simulink model "Model_InterpretationEngine64"  (R2022b)
settings: Solver=FixedStepDiscrete  StartTime=0.0  StopTime=5  RelTol=1e-3  EnableMultiTasking=on
InitFcn:
  | % Initialize model
  | ModelSettings=BTConfig.GetModelSettings();
  | 
  | ModelSettings.Validate();
  | 
  | ModelInit;
  | 
  | 
  | % load library data
  | GainLibrary_data;
  | % Load saved values from partition process
  | CapturedConstMask.LoadMapFromFile(bdroot)
  | % Load saved values from partition process
  | TSP_Mask.LoadMapFromFile(bdroot)
StartFcn:
  | % make sure all the simulated RTC requests are found
  | %RTC_SIM_OBJ.ValidateREQs();
undefined symbols (not defined in the file or in its folder): NumHFRefBPF, NumHFRefLPF
libraries: StateVar x112, TSP x56, FeaturePath x24
(part 4 of 5)

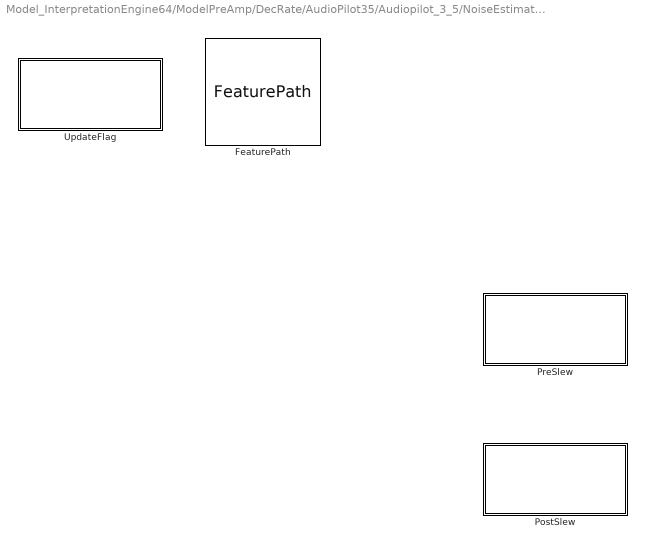
== system Model_InterpretationEngine64/ModelPreAmp/DecRate/AudioPilot35/Audiopilot_3_5/NoiseEstimationVariant/RegularNoiseEstimation/RatioCalculation ==
  FeaturePath : FeaturePath/FeaturePath  FeatureName=Ratio  IsGroup=off  GroupNumber=-1  IsModule=off  TriggerInit=[735 -166 850 -59]
      settings: SourceProductName=Bose Talaria
  PostSlew : Subsystem  mask(Talaria Target State Variable){TriggerInit=[1015 241 1155 309], TspName=PostSlew, StateName=PostSlew, UseSameName=on, IfdefMacro=[]}
      mask prompts: TriggerInit "Hidden: MoveFcn redraw"; TspName "Name:"; StateName "Name of StateVar:"; UseSameName "Use same name for state variable and TSP"; IfdefMacro "Additional #ifdef macro to enable trigger capture:"
      mask help: The TargetStateVar block encapsultes a Target State Probe (TSP), a State Variable, and a Trivial Interpretation between them.
      mask init:
      | [ok,tspPath,activeStatePath] = TargetStateVarMask.Init(gcbh);
      settings: MoveFcn=TargetStateVarMask.CB_TriggerInit(gcbh);
      mask Help: See help for StateVar and TSP blocks
      mask Callback TriggerInit: TargetStateVarMask.CB_TriggerInit(gcbh);
      mask TypeOptions TspName: TSP/TspName
      mask TypeOptions StateName: StateVar/StateName
      mask Callback UseSameName: TargetStateVarMask.CB_UseSameName(gcbh);
      mask TypeOptions IfdefMacro: TSP/IfdefMacro
      mask DialogControl AdvancedPanel Prompt: Advanced
      mask DialogControl ConvertToFullInterpretation Prompt: Irreversible conversion to full interpretation
      mask DialogControl ConvertToFullInterpretation Callback: TargetStateVarMask.CB_ConvertToFullInterpretation(gcbh);
      mask DialogControl ErrorContainer Prompt: Error Messages
      mask DialogControl ErrorText Prompt: The interpreted StateVar value is not yet available
      mask DialogControl TspPathText Prompt: TSP: Current parameter name: [AudiopilotRatioPostSlew]
      mask Display:
      | % retrieve icon definition
      | [path,w,h] = TargetStateVarMask.Icon();
      | 
      | % retrieve the block's pixel size
      | pos = get(gcbh,'position');
      | bw = pos(3) - pos(1);
      | bh = pos(4) - pos(2);
      | 
      | % draw centered icon
      | xAdj = bw/2 - w/2 + 5;
      | yAdj = bh/2 - h/2 + 4;
      | for i=1:length(path)
      | 	patch(path(i).x+xAdj, path(i).y+yAdj, path(i).rgb);
      | end
      | 
      | % show the top name or an X
      | if (exist('ok','var') && ok)
      | 	text(bw*0.5, bh*0.2, tspPath, 'horizontalAlignment', 'center');
      | 	patch(0,0,[1 1 1]);
      | 	patch(bw,bh,[1 1 1]);
      | else
      | 	tx=bw*0.03;
      | 	ty=bh*0.03;
      | 	patch([0 tx bw bw-tx], [ty 0 bh-ty bh], [1 0 0]);
      | 	patch([0 bw-tx bw tx], [bh-ty 0 ty bh], [1 0 0]);
      | end
  PreSlew : Subsystem  mask(Talaria Target State Variable){TriggerInit=[1015 91 1155 159], TspName=PreSlew, StateName=PreSlew, UseSameName=on, IfdefMacro=[]}
      mask prompts: TriggerInit "Hidden: MoveFcn redraw"; TspName "Name:"; StateName "Name of StateVar:"; UseSameName "Use same name for state variable and TSP"; IfdefMacro "Additional #ifdef macro to enable trigger capture:"
      mask help: The TargetStateVar block encapsultes a Target State Probe (TSP), a State Variable, and a Trivial Interpretation between them.
      mask init:
      | [ok,tspPath,activeStatePath] = TargetStateVarMask.Init(gcbh);
      settings: MoveFcn=TargetStateVarMask.CB_TriggerInit(gcbh);
      mask Help: See help for StateVar and TSP blocks
      mask Callback TriggerInit: TargetStateVarMask.CB_TriggerInit(gcbh);
      mask TypeOptions TspName: TSP/TspName
      mask TypeOptions StateName: StateVar/StateName
      mask Callback UseSameName: TargetStateVarMask.CB_UseSameName(gcbh);
      mask TypeOptions IfdefMacro: TSP/IfdefMacro
      mask DialogControl AdvancedPanel Prompt: Advanced
      mask DialogControl ConvertToFullInterpretation Prompt: Irreversible conversion to full interpretation
      mask DialogControl ConvertToFullInterpretation Callback: TargetStateVarMask.CB_ConvertToFullInterpretation(gcbh);
      mask DialogControl ErrorContainer Prompt: Error Messages
      mask DialogControl ErrorText Prompt: The interpreted StateVar value is not yet available
      mask DialogControl TspPathText Prompt: TSP: Current parameter name: [AudiopilotRatioPreSlew]
      mask Display:
      | % retrieve icon definition
      | [path,w,h] = TargetStateVarMask.Icon();
      | 
      | % retrieve the block's pixel size
      | pos = get(gcbh,'position');
      | bw = pos(3) - pos(1);
      | bh = pos(4) - pos(2);
      | 
      | % draw centered icon
      | xAdj = bw/2 - w/2 + 5;
      | yAdj = bh/2 - h/2 + 4;
      | for i=1:length(path)
      | 	patch(path(i).x+xAdj, path(i).y+yAdj, path(i).rgb);
      | end
      | 
      | % show the top name or an X
      | if (exist('ok','var') && ok)
      | 	text(bw*0.5, bh*0.2, tspPath, 'horizontalAlignment', 'center');
      | 	patch(0,0,[1 1 1]);
      | 	patch(bw,bh,[1 1 1]);
      | else
      | 	tx=bw*0.03;
      | 	ty=bh*0.03;
      | 	patch([0 tx bw bw-tx], [ty 0 bh-ty bh], [1 0 0]);
      | 	patch([0 bw-tx bw tx], [bh-ty 0 ty bh], [1 0 0]);
      | end
  UpdateFlag : Subsystem  mask(Talaria Target State Variable){TriggerInit=[550 -144 690 -76], TspName=UpdateFlag, StateName=UpdateFlag, UseSameName=on, IfdefMacro=[]}
      mask prompts: TriggerInit "Hidden: MoveFcn redraw"; TspName "Name:"; StateName "Name of StateVar:"; UseSameName "Use same name for state variable and TSP"; IfdefMacro "Additional #ifdef macro to enable trigger capture:"
      mask help: The TargetStateVar block encapsultes a Target State Probe (TSP), a State Variable, and a Trivial Interpretation between them.
      mask init:
      | [ok,tspPath,activeStatePath] = TargetStateVarMask.Init(gcbh);
      settings: MoveFcn=TargetStateVarMask.CB_TriggerInit(gcbh);
      mask Help: See help for StateVar and TSP blocks
      mask Callback TriggerInit: TargetStateVarMask.CB_TriggerInit(gcbh);
      mask TypeOptions TspName: TSP/TspName
      mask TypeOptions StateName: StateVar/StateName
      mask Callback UseSameName: TargetStateVarMask.CB_UseSameName(gcbh);
      mask TypeOptions IfdefMacro: TSP/IfdefMacro
      mask DialogControl AdvancedPanel Prompt: Advanced
      mask DialogControl ConvertToFullInterpretation Prompt: Irreversible conversion to full interpretation
      mask DialogControl ConvertToFullInterpretation Callback: TargetStateVarMask.CB_ConvertToFullInterpretation(gcbh);
      mask DialogControl ErrorContainer Prompt: Error Messages
      mask DialogControl ErrorText Prompt: The interpreted StateVar value is not yet available
      mask DialogControl TspPathText Prompt: TSP: Current parameter name: [AudiopilotRatioUpdateFlag]
      mask Display:
      | % retrieve icon definition
      | [path,w,h] = TargetStateVarMask.Icon();
      | 
      | % retrieve the block's pixel size
      | pos = get(gcbh,'position');
      | bw = pos(3) - pos(1);
      | bh = pos(4) - pos(2);
      | 
      | % draw centered icon
      | xAdj = bw/2 - w/2 + 5;
      | yAdj = bh/2 - h/2 + 4;
      | for i=1:length(path)
      | 	patch(path(i).x+xAdj, path(i).y+yAdj, path(i).rgb);
      | end
      | 
      | % show the top name or an X
      | if (exist('ok','var') && ok)
      | 	text(bw*0.5, bh*0.2, tspPath, 'horizontalAlignment', 'center');
      | 	patch(0,0,[1 1 1]);
      | 	patch(bw,bh,[1 1 1]);
      | else
      | 	tx=bw*0.03;
      | 	ty=bh*0.03;
      | 	patch([0 tx bw bw-tx], [ty 0 bh-ty bh], [1 0 0]);
      | 	patch([0 bw-tx bw tx], [bh-ty 0 ty bh], [1 0 0]);
      | end

== system Model_InterpretationEngine64/ModelPreAmp/DecRate/AudioPilot35/EntertainmentLevelDetection/AudiopilotLevelDetect/Monitor/env ==
  StateVar : StateVar/StateVar  TriggerInit=[490 139 605 201]  StateName=EnvDb
      settings: SourceProductName=Bose Talaria
  TSP : TSP/TSP  TriggerInit=[110 134 215 206]  TspName=EnvDb  IfDefMacro=IfdefMacro  Role=Automatic
      settings: SourceProductName=Bose Talaria
  TrivialInterpretation : StateVar/TrivialInterpretation  TriggerInit=[330 148 380 192]
      settings: SourceProductName=Bose Talaria
  wires:
  TrivialInterpretation/1 -> StateVar/1
  TSP/1 -> TrivialInterpretation/1

== system Model_InterpretationEngine64/ModelPreAmp/DecRate/AudioPilot35/EntertainmentLevelDetection/AudiopilotLevelDetect/Monitor/level ==
  StateVar : StateVar/StateVar  TriggerInit=[490 139 605 201]  StateName=LevelDbspl
      settings: SourceProductName=Bose Talaria
  TSP : TSP/TSP  TriggerInit=[110 134 215 206]  TspName=LevelDbspl  IfDefMacro=IfdefMacro  Role=Automatic
      settings: SourceProductName=Bose Talaria
  TrivialInterpretation : StateVar/TrivialInterpretation  TriggerInit=[330 148 380 192]
      settings: SourceProductName=Bose Talaria
  wires:
  TrivialInterpretation/1 -> StateVar/1
  TSP/1 -> TrivialInterpretation/1

== system Model_InterpretationEngine64/ModelPreAmp/DecRate/AudioPilot35/EntertainmentLevelDetection/DyneqLevelDetect/Monitor/env ==
  StateVar : StateVar/StateVar  TriggerInit=[490 139 605 201]  StateName=EnvDb
      settings: SourceProductName=Bose Talaria
  TSP : TSP/TSP  TriggerInit=[110 134 215 206]  TspName=EnvDb  IfDefMacro=IfdefMacro  Role=Automatic
      settings: SourceProductName=Bose Talaria
  TrivialInterpretation : StateVar/TrivialInterpretation  TriggerInit=[330 148 380 192]
      settings: SourceProductName=Bose Talaria
  wires:
  TrivialInterpretation/1 -> StateVar/1
  TSP/1 -> TrivialInterpretation/1

== system Model_InterpretationEngine64/ModelPreAmp/DecRate/AudioPilot35/EntertainmentLevelDetection/DyneqLevelDetect/Monitor/level ==
  StateVar : StateVar/StateVar  TriggerInit=[490 139 605 201]  StateName=LevelDbspl
      settings: SourceProductName=Bose Talaria
  TSP : TSP/TSP  TriggerInit=[110 134 215 206]  TspName=LevelDbspl  IfDefMacro=IfdefMacro  Role=Automatic
      settings: SourceProductName=Bose Talaria
  TrivialInterpretation : StateVar/TrivialInterpretation  TriggerInit=[330 148 380 192]
      settings: SourceProductName=Bose Talaria
  wires:
  TrivialInterpretation/1 -> StateVar/1
  TSP/1 -> TrivialInterpretation/1

== system Model_InterpretationEngine64/ModelPreAmp/DecRate/Medusa5H1/MedusaHoligram/Medusa5H1 Part 1/CAE Treble Boost/Audio Passthrough ==
  Target StateVar : Subsystem  mask(Talaria Target State Variable){TriggerInit=[235 166 375 234], TspName=DummyState, StateName=DummyState, UseSameName=on, IfdefMacro=[]}
      mask prompts: TriggerInit "Hidden: MoveFcn redraw"; TspName "Name:"; StateName "Name of StateVar:"; UseSameName "Use same name for state variable and TSP"; IfdefMacro "Additional #ifdef macro to enable trigger capture:"
      mask help: The TargetStateVar block encapsultes a Target State Probe (TSP), a State Variable, and a Trivial Interpretation between them.
      mask init:
      | [ok,tspPath,activeStatePath] = TargetStateVarMask.Init(gcbh);
      settings: MoveFcn=TargetStateVarMask.CB_TriggerInit(gcbh);
      mask Help: See help for StateVar and TSP blocks
      mask Callback TriggerInit: TargetStateVarMask.CB_TriggerInit(gcbh);
      mask TypeOptions TspName: TSP/TspName
      mask TypeOptions StateName: StateVar/StateName
      mask Callback UseSameName: TargetStateVarMask.CB_UseSameName(gcbh);
      mask TypeOptions IfdefMacro: TSP/IfdefMacro
      mask DialogControl AdvancedPanel Prompt: Advanced
      mask DialogControl ConvertToFullInterpretation Prompt: Irreversible conversion to full interpretation
      mask DialogControl ConvertToFullInterpretation Callback: TargetStateVarMask.CB_ConvertToFullInterpretation(gcbh);
      mask DialogControl ErrorContainer Prompt: Error Messages
      mask DialogControl ErrorText Prompt: The interpreted StateVar value is not yet available
      mask DialogControl TspPathText Prompt: TSP: Current parameter name: [PreAmpMedusaDummyState]
      mask Display:
      | % retrieve icon definition
      | [path,w,h] = TargetStateVarMask.Icon();
      | 
      | % retrieve the block's pixel size
      | pos = get(gcbh,'position');
      | bw = pos(3) - pos(1);
      | bh = pos(4) - pos(2);
      | 
      | % draw centered icon
      | xAdj = bw/2 - w/2 + 5;
      | yAdj = bh/2 - h/2 + 4;
      | for i=1:length(path)
      | 	patch(path(i).x+xAdj, path(i).y+yAdj, path(i).rgb);
      | end
      | 
      | % show the top name or an X
      | if (exist('ok','var') && ok)
      | 	text(bw*0.5, bh*0.2, tspPath, 'horizontalAlignment', 'center');
      | 	patch(0,0,[1 1 1]);
      | 	patch(bw,bh,[1 1 1]);
      | else
      | 	tx=bw*0.03;
      | 	ty=bh*0.03;
      | 	patch([0 tx bw bw-tx], [ty 0 bh-ty bh], [1 0 0]);
      | 	patch([0 bw-tx bw tx], [bh-ty 0 ty bh], [1 0 0]);
      | end

== system Model_InterpretationEngine64/ModelPreAmp/DecRate/Medusa5H1/MedusaHoligram/Medusa5H1 Part 1/CAE Treble Boost/CAE Treble Boost ==

== system Model_InterpretationEngine64/ModelPreAmp/DecRate/Medusa5H1/MedusaHoligram/Medusa5H1 Part 2/Mono Detector/Mono Detector ==
  Target StateVar : Subsystem  mask(Talaria Target State Variable){TriggerInit=[875 1951 1015 2019], TspName=LevelCenter, StateName=LevelCenter, UseSameName=on, IfdefMacro=[]}
      mask prompts: TriggerInit "Hidden: MoveFcn redraw"; TspName "Name:"; StateName "Name of StateVar:"; UseSameName "Use same name for state variable and TSP"; IfdefMacro "Additional #ifdef macro to enable trigger capture:"
      mask help: The TargetStateVar block encapsultes a Target State Probe (TSP), a State Variable, and a Trivial Interpretation between them.
      mask init:
      | [ok,tspPath,activeStatePath] = TargetStateVarMask.Init(gcbh);
      settings: MoveFcn=TargetStateVarMask.CB_TriggerInit(gcbh);
      mask Help: See help for StateVar and TSP blocks
      mask Callback TriggerInit: TargetStateVarMask.CB_TriggerInit(gcbh);
      mask TypeOptions TspName: TSP/TspName
      mask TypeOptions StateName: StateVar/StateName
      mask Callback UseSameName: TargetStateVarMask.CB_UseSameName(gcbh);
      mask TypeOptions IfdefMacro: TSP/IfdefMacro
      mask DialogControl AdvancedPanel Prompt: Advanced
      mask DialogControl ConvertToFullInterpretation Prompt: Irreversible conversion to full interpretation
      mask DialogControl ConvertToFullInterpretation Callback: TargetStateVarMask.CB_ConvertToFullInterpretation(gcbh);
      mask DialogControl ErrorContainer Prompt: Error Messages
      mask DialogControl ErrorText Prompt: The interpreted StateVar value is not yet available
      mask DialogControl TspPathText Prompt: TSP: Current parameter name: [PreAmpMedusaMonoDetectorLevelCenter]
      mask Display:
      | % retrieve icon definition
      | [path,w,h] = TargetStateVarMask.Icon();
      | 
      | % retrieve the block's pixel size
      | pos = get(gcbh,'position');
      | bw = pos(3) - pos(1);
      | bh = pos(4) - pos(2);
      | 
      | % draw centered icon
      | xAdj = bw/2 - w/2 + 5;
      | yAdj = bh/2 - h/2 + 4;
      | for i=1:length(path)
      | 	patch(path(i).x+xAdj, path(i).y+yAdj, path(i).rgb);
      | end
      | 
      | % show the top name or an X
      | if (exist('ok','var') && ok)
      | 	text(bw*0.5, bh*0.2, tspPath, 'horizontalAlignment', 'center');
      | 	patch(0,0,[1 1 1]);
      | 	patch(bw,bh,[1 1 1]);
      | else
      | 	tx=bw*0.03;
      | 	ty=bh*0.03;
      | 	patch([0 tx bw bw-tx], [ty 0 bh-ty bh], [1 0 0]);
      | 	patch([0 bw-tx bw tx], [bh-ty 0 ty bh], [1 0 0]);
      | end

== system Model_InterpretationEngine64/ModelPreAmp/DecRate/Medusa5H1/MedusaHoligram/Medusa5H1 Part 2/Mono Detector/Target StateVar ==
  StateVar : StateVar/StateVar  TriggerInit=[490 139 605 201]  StateName=IsStereo
      settings: SourceProductName=Bose Talaria
  TSP : TSP/TSP  TriggerInit=[110 134 215 206]  TspName=IsStereo  IfDefMacro=IfdefMacro  Role=Automatic
      settings: SourceProductName=Bose Talaria
  TrivialInterpretation : StateVar/TrivialInterpretation  TriggerInit=[330 148 380 192]
      settings: SourceProductName=Bose Talaria
  wires:
  TrivialInterpretation/1 -> StateVar/1
  TSP/1 -> TrivialInterpretation/1

== system Model_InterpretationEngine64/ModelPreAmp/DecRate/Medusa5H1/MedusaHoligram/Medusa5H1 Part 2/Mono Detector/Target StateVar1 ==
  StateVar : StateVar/StateVar  TriggerInit=[490 139 605 201]  StateName=IsActive
      settings: SourceProductName=Bose Talaria
  TSP : TSP/TSP  TriggerInit=[110 134 215 206]  TspName=IsActive  IfDefMacro=IfdefMacro  Role=Automatic
      settings: SourceProductName=Bose Talaria
  TrivialInterpretation : StateVar/TrivialInterpretation  TriggerInit=[330 148 380 192]
      settings: SourceProductName=Bose Talaria
  wires:
  TrivialInterpretation/1 -> StateVar/1
  TSP/1 -> TrivialInterpretation/1

== system Model_InterpretationEngine64/NEAR/Near1p1/VolumeMute/VolMuteCh1/Ann1NonEntGainCalc/boost/Target StateVar ==
  StateVar : StateVar/StateVar  TriggerInit=[490 139 605 201]  StateName=GetNonEntBoostLeveldB
      settings: SourceProductName=Bose Talaria
  TSP : TSP/TSP  TriggerInit=[110 134 215 206]  TspName=GetNonEntBoostLeveldB  IfDefMacro=IfdefMacro  Role=Automatic
      settings: SourceProductName=Bose Talaria
  TrivialInterpretation : StateVar/TrivialInterpretation  TriggerInit=[330 148 380 192]
      settings: SourceProductName=Bose Talaria
  wires:
  TrivialInterpretation/1 -> StateVar/1
  TSP/1 -> TrivialInterpretation/1

== system Model_InterpretationEngine64/NEAR/Near1p1/VolumeMute/VolMuteCh2/Ann2NonEntGainCalc/boost/Target StateVar ==
  StateVar : StateVar/StateVar  TriggerInit=[490 139 605 201]  StateName=GetNonEntBoostLeveldB
      settings: SourceProductName=Bose Talaria
  TSP : TSP/TSP  TriggerInit=[110 134 215 206]  TspName=GetNonEntBoostLeveldB  IfDefMacro=IfdefMacro  Role=Automatic
      settings: SourceProductName=Bose Talaria
  TrivialInterpretation : StateVar/TrivialInterpretation  TriggerInit=[330 148 380 192]
      settings: SourceProductName=Bose Talaria
  wires:
  TrivialInterpretation/1 -> StateVar/1
  TSP/1 -> TrivialInterpretation/1

== system Model_InterpretationEngine64/NEAR/Near1p1/VolumeMute/VolMuteCh3/Ann3NonEntGainCalc/boost/Target StateVar ==
  StateVar : StateVar/StateVar  TriggerInit=[490 139 605 201]  StateName=GetNonEntBoostLeveldB
      settings: SourceProductName=Bose Talaria
  TSP : TSP/TSP  TriggerInit=[110 134 215 206]  TspName=GetNonEntBoostLeveldB  IfDefMacro=IfdefMacro  Role=Automatic
      settings: SourceProductName=Bose Talaria
  TrivialInterpretation : StateVar/TrivialInterpretation  TriggerInit=[330 148 380 192]
      settings: SourceProductName=Bose Talaria
  wires:
  TrivialInterpretation/1 -> StateVar/1
  TSP/1 -> TrivialInterpretation/1

== system Model_InterpretationEngine64/NEAR/Near1p1/VolumeMute/VolMuteCh4/Ann4NonEntGainCalc/boost/Target StateVar ==
  StateVar : StateVar/StateVar  TriggerInit=[490 139 605 201]  StateName=GetNonEntBoostLeveldB
      settings: SourceProductName=Bose Talaria
  TSP : TSP/TSP  TriggerInit=[110 134 215 206]  TspName=GetNonEntBoostLeveldB  IfDefMacro=IfdefMacro  Role=Automatic
      settings: SourceProductName=Bose Talaria
  TrivialInterpretation : StateVar/TrivialInterpretation  TriggerInit=[330 148 380 192]
      settings: SourceProductName=Bose Talaria
  wires:
  TrivialInterpretation/1 -> StateVar/1
  TSP/1 -> TrivialInterpretation/1

== system Model_InterpretationEngine64/ModelPreAmp/DecRate/AudioPilot35/Audiopilot_3_5/NoiseEstimationVariant/RegularNoiseEstimation/HFNoiseEstimatorCoh/HfNoiseMusicSeparation  ==
  note: Optimization Idea:
      | 1. Use 1-D array to store HALF 3-D GXY matrix, saving 16 KB
  MicPsdLevel : Subsystem
  NoisePsdLevel : Subsystem

== system Model_InterpretationEngine64/ModelPreAmp/DecRate/AudioPilot35/Audiopilot_3_5/NoiseEstimationVariant/RegularNoiseEstimation/HFNoiseEstimatorCoh/PostProcessing ==
  HfImpulseRejection : Subsystem
  PostSlew : Subsystem  mask(Talaria Target State Variable){TriggerInit=[735 161 875 229], TspName=PostSlew, StateName=PostSlew, UseSameName=on, IfdefMacro=[]}
      mask prompts: TriggerInit "Hidden: MoveFcn redraw"; TspName "Name:"; StateName "Name of StateVar:"; UseSameName "Use same name for state variable and TSP"; IfdefMacro "Additional #ifdef macro to enable trigger capture:"
      mask help: The TargetStateVar block encapsultes a Target State Probe (TSP), a State Variable, and a Trivial Interpretation between them.
      mask init:
      | [ok,tspPath,activeStatePath] = TargetStateVarMask.Init(gcbh);
      settings: MoveFcn=TargetStateVarMask.CB_TriggerInit(gcbh);
      mask Help: See help for StateVar and TSP blocks
      mask Callback TriggerInit: TargetStateVarMask.CB_TriggerInit(gcbh);
      mask TypeOptions TspName: TSP/TspName
      mask TypeOptions StateName: StateVar/StateName
      mask Callback UseSameName: TargetStateVarMask.CB_UseSameName(gcbh);
      mask TypeOptions IfdefMacro: TSP/IfdefMacro
      mask DialogControl AdvancedPanel Prompt: Advanced
      mask DialogControl ConvertToFullInterpretation Prompt: Irreversible conversion to full interpretation
      mask DialogControl ConvertToFullInterpretation Callback: TargetStateVarMask.CB_ConvertToFullInterpretation(gcbh);
      mask DialogControl ErrorContainer Prompt: Error Messages
      mask Display:
      | % retrieve icon definition
      | [path,w,h] = TargetStateVarMask.Icon();
      | 
      | % retrieve the block's pixel size
      | pos = get(gcbh,'position');
      | bw = pos(3) - pos(1);
      | bh = pos(4) - pos(2);
      | 
      | % draw centered icon
      | xAdj = bw/2 - w/2 + 5;
      | yAdj = bh/2 - h/2 + 4;
      | for i=1:length(path)
      | 	patch(path(i).x+xAdj, path(i).y+yAdj, path(i).rgb);
      | end
      | 
      | % show the top name or an X
      | if (exist('ok','var') && ok)
      | 	text(bw*0.5, bh*0.2, tspPath, 'horizontalAlignment', 'center');
      | 	patch(0,0,[1 1 1]);
      | 	patch(bw,bh,[1 1 1]);
      | else
      | 	tx=bw*0.03;
      | 	ty=bh*0.03;
      | 	patch([0 tx bw bw-tx], [ty 0 bh-ty bh], [1 0 0]);
      | 	patch([0 bw-tx bw tx], [bh-ty 0 ty bh], [1 0 0]);
      | end
  PreSlew : Subsystem  mask(Talaria Target State Variable){TriggerInit=[735 251 875 319], TspName=PreSlew, StateName=PreSlew, UseSameName=on, IfdefMacro=[]}
      mask prompts: TriggerInit "Hidden: MoveFcn redraw"; TspName "Name:"; StateName "Name of StateVar:"; UseSameName "Use same name for state variable and TSP"; IfdefMacro "Additional #ifdef macro to enable trigger capture:"
      mask help: The TargetStateVar block encapsultes a Target State Probe (TSP), a State Variable, and a Trivial Interpretation between them.
      mask init:
      | [ok,tspPath,activeStatePath] = TargetStateVarMask.Init(gcbh);
      settings: MoveFcn=TargetStateVarMask.CB_TriggerInit(gcbh);
      mask Help: See help for StateVar and TSP blocks
      mask Callback TriggerInit: TargetStateVarMask.CB_TriggerInit(gcbh);
      mask TypeOptions TspName: TSP/TspName
      mask TypeOptions StateName: StateVar/StateName
      mask Callback UseSameName: TargetStateVarMask.CB_UseSameName(gcbh);
      mask TypeOptions IfdefMacro: TSP/IfdefMacro
      mask DialogControl AdvancedPanel Prompt: Advanced
      mask DialogControl ConvertToFullInterpretation Prompt: Irreversible conversion to full interpretation
      mask DialogControl ConvertToFullInterpretation Callback: TargetStateVarMask.CB_ConvertToFullInterpretation(gcbh);
      mask DialogControl ErrorContainer Prompt: Error Messages
      mask Display:
      | % retrieve icon definition
      | [path,w,h] = TargetStateVarMask.Icon();
      | 
      | % retrieve the block's pixel size
      | pos = get(gcbh,'position');
      | bw = pos(3) - pos(1);
      | bh = pos(4) - pos(2);
      | 
      | % draw centered icon
      | xAdj = bw/2 - w/2 + 5;
      | yAdj = bh/2 - h/2 + 4;
      | for i=1:length(path)
      | 	patch(path(i).x+xAdj, path(i).y+yAdj, path(i).rgb);
      | end
      | 
      | % show the top name or an X
      | if (exist('ok','var') && ok)
      | 	text(bw*0.5, bh*0.2, tspPath, 'horizontalAlignment', 'center');
      | 	patch(0,0,[1 1 1]);
      | 	patch(bw,bh,[1 1 1]);
      | else
      | 	tx=bw*0.03;
      | 	ty=bh*0.03;
      | 	patch([0 tx bw bw-tx], [ty 0 bh-ty bh], [1 0 0]);
      | 	patch([0 bw-tx bw tx], [bh-ty 0 ty bh], [1 0 0]);
      | end

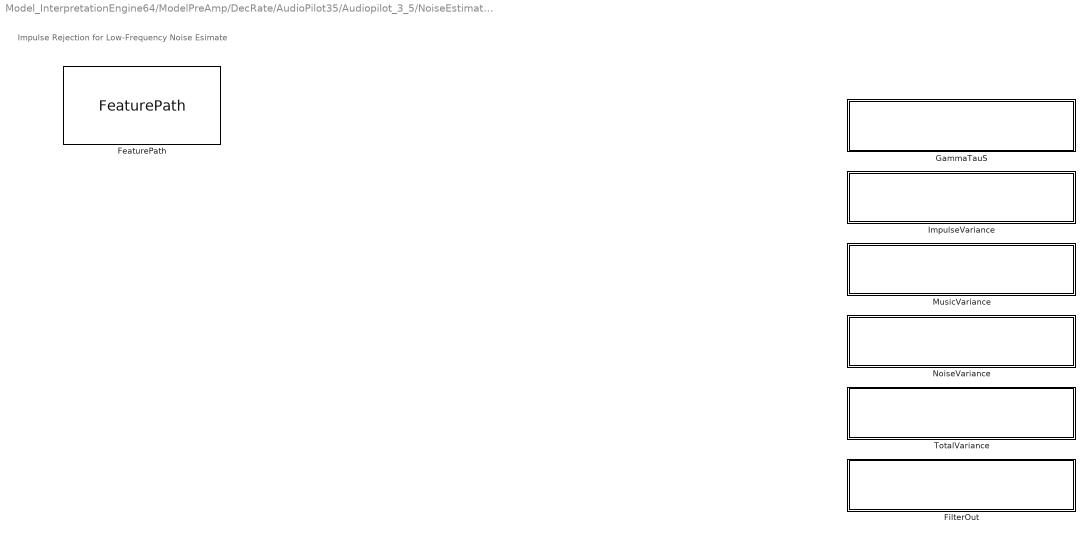
== system Model_InterpretationEngine64/ModelPreAmp/DecRate/AudioPilot35/Audiopilot_3_5/NoiseEstimationVariant/RegularNoiseEstimation/LFNoiseEstimatorCoh/LfNoiseImpulseRejection ==
  note: Impulse Rejection for Low-Frequency Noise Esimate
  FeaturePath : FeaturePath/FeaturePath  FeatureName=ImpulseRejection  IsGroup=off  GroupNumber=-1  IsModule=off  TriggerInit=[-70 349 105 436]
      settings: SourceProductName=Bose Talaria
  FilterOut : Subsystem  mask(Talaria Target State Variable){TriggerInit=[805 788 1055 842], TspName=FilterOut, StateName=FilterOut, UseSameName=on, IfdefMacro=[]}
      mask prompts: TriggerInit "Hidden: MoveFcn redraw"; TspName "Name:"; StateName "Name of StateVar:"; UseSameName "Use same name for state variable and TSP"; IfdefMacro "Additional #ifdef macro to enable trigger capture:"
      mask help: The TargetStateVar block encapsultes a Target State Probe (TSP), a State Variable, and a Trivial Interpretation between them.
      mask init:
      | [ok,tspPath,activeStatePath] = TargetStateVarMask.Init(gcbh);
      settings: MoveFcn=TargetStateVarMask.CB_TriggerInit(gcbh);
      mask Help: See help for StateVar and TSP blocks
      mask Callback TriggerInit: TargetStateVarMask.CB_TriggerInit(gcbh);
      mask TypeOptions TspName: TSP/TspName
      mask TypeOptions StateName: StateVar/StateName
      mask Callback UseSameName: TargetStateVarMask.CB_UseSameName(gcbh);
      mask TypeOptions IfdefMacro: TSP/IfdefMacro
      mask DialogControl AdvancedPanel Prompt: Advanced
      mask DialogControl ConvertToFullInterpretation Prompt: Irreversible conversion to full interpretation
      mask DialogControl ConvertToFullInterpretation Callback: TargetStateVarMask.CB_ConvertToFullInterpretation(gcbh);
      mask DialogControl ErrorContainer Prompt: Error Messages
      mask DialogControl ErrorText Prompt: The interpreted StateVar value is not yet available
      mask DialogControl TspPathText Prompt: TSP: Current parameter name: [AudiopilotLfNoiseImpulseRejectionFilterOut]
      mask Display:
      | % retrieve icon definition
      | [path,w,h] = TargetStateVarMask.Icon();
      | 
      | % retrieve the block's pixel size
      | pos = get(gcbh,'position');
      | bw = pos(3) - pos(1);
      | bh = pos(4) - pos(2);
      | 
      | % draw centered icon
      | xAdj = bw/2 - w/2 + 5;
      | yAdj = bh/2 - h/2 + 4;
      | for i=1:length(path)
      | 	patch(path(i).x+xAdj, path(i).y+yAdj, path(i).rgb);
      | end
      | 
      | % show the top name or an X
      | if (exist('ok','var') && ok)
      | 	text(bw*0.5, bh*0.2, tspPath, 'horizontalAlignment', 'center');
      | 	patch(0,0,[1 1 1]);
      | 	patch(bw,bh,[1 1 1]);
      | else
      | 	tx=bw*0.03;
      | 	ty=bh*0.03;
      | 	patch([0 tx bw bw-tx], [ty 0 bh-ty bh], [1 0 0]);
      | 	patch([0 bw-tx bw tx], [bh-ty 0 ty bh], [1 0 0]);
      | end
  GammaTauS : Subsystem
  ImpulseVariance : Subsystem
  MusicVariance : Subsystem
  NoiseVariance : Subsystem
  TotalVariance : Subsystem

== system Model_InterpretationEngine64/ModelPreAmp/DecRate/AudioPilot35/Audiopilot_3_5/NoiseEstimationVariant/RegularNoiseEstimation/LFNoiseEstimatorCoh/MicLevel ==
  StateVar : StateVar/StateVar  TriggerInit=[490 139 605 201]  StateName=MicLevel
      settings: SourceProductName=Bose Talaria
  TSP : TSP/TSP  TriggerInit=[110 134 215 206]  TspName=MicLevel  IfDefMacro=IfdefMacro  Role=Automatic
      settings: SourceProductName=Bose Talaria
  TrivialInterpretation : StateVar/TrivialInterpretation  TriggerInit=[330 148 380 192]
      settings: SourceProductName=Bose Talaria
  wires:
  TSP/1 -> TrivialInterpretation/1
  TrivialInterpretation/1 -> StateVar/1

== system Model_InterpretationEngine64/ModelPreAmp/DecRate/AudioPilot35/Audiopilot_3_5/NoiseEstimationVariant/RegularNoiseEstimation/LFNoiseEstimatorCoh/MicOut ==
  StateVar : StateVar/StateVar  TriggerInit=[490 139 605 201]  StateName=MicOut
      settings: SourceProductName=Bose Talaria
  TSP : TSP/TSP  TriggerInit=[110 134 215 206]  TspName=MicOut  IfDefMacro=IfdefMacro  Role=Automatic
      settings: SourceProductName=Bose Talaria
  TrivialInterpretation : StateVar/TrivialInterpretation  TriggerInit=[330 148 380 192]
      settings: SourceProductName=Bose Talaria
  wires:
  TSP/1 -> TrivialInterpretation/1
  TrivialInterpretation/1 -> StateVar/1

== system Model_InterpretationEngine64/ModelPreAmp/DecRate/AudioPilot35/Audiopilot_3_5/NoiseEstimationVariant/RegularNoiseEstimation/LFNoiseEstimatorCoh/MusicOut ==
  StateVar : StateVar/StateVar  TriggerInit=[490 139 605 201]  StateName=MusicOut
      settings: SourceProductName=Bose Talaria
  TSP : TSP/TSP  TriggerInit=[110 134 215 206]  TspName=MusicOut  IfDefMacro=IfdefMacro  Role=Automatic
      settings: SourceProductName=Bose Talaria
  TrivialInterpretation : StateVar/TrivialInterpretation  TriggerInit=[330 148 380 192]
      settings: SourceProductName=Bose Talaria
  wires:
  TSP/1 -> TrivialInterpretation/1
  TrivialInterpretation/1 -> StateVar/1

== system Model_InterpretationEngine64/ModelPreAmp/DecRate/AudioPilot35/Audiopilot_3_5/NoiseEstimationVariant/RegularNoiseEstimation/LFNoiseEstimatorCoh/NoiseOut ==
  StateVar : StateVar/StateVar  TriggerInit=[490 139 605 201]  StateName=NoiseOut
      settings: SourceProductName=Bose Talaria
  TSP : TSP/TSP  TriggerInit=[110 134 215 206]  TspName=NoiseOut  IfDefMacro=IfdefMacro  Role=Automatic
      settings: SourceProductName=Bose Talaria
  TrivialInterpretation : StateVar/TrivialInterpretation  TriggerInit=[330 148 380 192]
      settings: SourceProductName=Bose Talaria
  wires:
  TSP/1 -> TrivialInterpretation/1
  TrivialInterpretation/1 -> StateVar/1

== system Model_InterpretationEngine64/ModelPreAmp/DecRate/AudioPilot35/Audiopilot_3_5/NoiseEstimationVariant/RegularNoiseEstimation/LFNoiseEstimatorCoh/PostSlew ==
  StateVar : StateVar/StateVar  TriggerInit=[490 139 605 201]  StateName=PostSlew
      settings: SourceProductName=Bose Talaria
  TSP : TSP/TSP  TriggerInit=[110 134 215 206]  TspName=PostSlew  IfDefMacro=IfdefMacro  Role=Automatic
      settings: SourceProductName=Bose Talaria
  TrivialInterpretation : StateVar/TrivialInterpretation  TriggerInit=[330 148 380 192]
      settings: SourceProductName=Bose Talaria
  wires:
  TSP/1 -> TrivialInterpretation/1
  TrivialInterpretation/1 -> StateVar/1

== system Model_InterpretationEngine64/ModelPreAmp/DecRate/AudioPilot35/Audiopilot_3_5/NoiseEstimationVariant/RegularNoiseEstimation/LFNoiseEstimatorCoh/PreSlew ==
  StateVar : StateVar/StateVar  TriggerInit=[490 139 605 201]  StateName=PreSlew
      settings: SourceProductName=Bose Talaria
  TSP : TSP/TSP  TriggerInit=[110 134 215 206]  TspName=PreSlew  IfDefMacro=IfdefMacro  Role=Automatic
      settings: SourceProductName=Bose Talaria
  TrivialInterpretation : StateVar/TrivialInterpretation  TriggerInit=[330 148 380 192]
      settings: SourceProductName=Bose Talaria
  wires:
  TSP/1 -> TrivialInterpretation/1
  TrivialInterpretation/1 -> StateVar/1

== system Model_InterpretationEngine64/ModelPreAmp/DecRate/AudioPilot35/Audiopilot_3_5/NoiseEstimationVariant/RegularNoiseEstimation/LFNoiseEstimatorCoh/PreSpeedBound ==
  StateVar : StateVar/StateVar  TriggerInit=[490 139 605 201]  StateName=PreSpeedBound
      settings: SourceProductName=Bose Talaria
  TSP : TSP/TSP  TriggerInit=[110 134 215 206]  TspName=PreSpeedBound  IfDefMacro=IfdefMacro  Role=Automatic
      settings: SourceProductName=Bose Talaria
  TrivialInterpretation : StateVar/TrivialInterpretation  TriggerInit=[330 148 380 192]
      settings: SourceProductName=Bose Talaria
  wires:
  TSP/1 -> TrivialInterpretation/1
  TrivialInterpretation/1 -> StateVar/1

== system Model_InterpretationEngine64/ModelPreAmp/DecRate/AudioPilot35/Audiopilot_3_5/NoiseEstimationVariant/RegularNoiseEstimation/LFNoiseEstimatorCoh/SpeedBoundsAndNoiseSlew ==
  SpeedBounds : Subsystem  mask(AudioPilot - Speed Bounds for Low Frequency Noise Estimate){FeatureName=SpeedBounds, Config=Config.SpeedBounds}
      mask prompts: FeatureName "Feature Name:"; Config "SpeedBoundsConfig"
      mask help: This block bounds the noise estimate with a minimum value and a maximum value, which are set based on the speed. The tables of speed bounds must each have a fixed number of entries (TableSize in BTC), but the indices can be irregularly spaced. This is specified by *_speed_bounds_axis. The minimum and maximum values are then correspondingly specified by *_speed_bounds_min_dbspl and *_speed_bounds_max_dbspl.
      mask init:
      | blkh = gcbh;
      | 
      | Config = BTConfig.Assert(blkh,Config);
      | Config.Validate();
      | 
      | BTConfig.InitSetFeatureIfPresent(blkh,'FeatureName');
      mask Help:
      | Arguments for this block:
      | 
      | Design Time Configuration
      | The Feature Name can be specified unless a BTC instance is used, in which case, the instance name will be used as Feature Name.
      | 
      | Build Time Configuration
      | The block can be configured using a object of class, SpeedBoundsConfig.
      mask TypeOptions FeatureName: FeaturePath/FeatureName
      mask Callback Config: BTConfig.CallbackHideIfPresent(gcbh,{'FeatureName'});
      mask DialogControl DTCTitle Prompt: <b> Design Time Configuration </b>
      mask DialogControl BTCTitle Prompt: <b> Build Time Configuration </b>

== system Model_InterpretationEngine64/ModelPreAmp/DecRate/AudioPilot35/Audiopilot_3_5/NoiseEstimationVariant/RegularNoiseEstimation/RatioCalculation/PostSlew ==
  StateVar : StateVar/StateVar  TriggerInit=[490 139 605 201]  StateName=PostSlew
      settings: SourceProductName=Bose Talaria
  TSP : TSP/TSP  TriggerInit=[110 134 215 206]  TspName=PostSlew  IfDefMacro=IfdefMacro  Role=Automatic
      settings: SourceProductName=Bose Talaria
  TrivialInterpretation : StateVar/TrivialInterpretation  TriggerInit=[330 148 380 192]
      settings: SourceProductName=Bose Talaria
  wires:
  TSP/1 -> TrivialInterpretation/1
  TrivialInterpretation/1 -> StateVar/1

== system Model_InterpretationEngine64/ModelPreAmp/DecRate/AudioPilot35/Audiopilot_3_5/NoiseEstimationVariant/RegularNoiseEstimation/RatioCalculation/PreSlew ==
  StateVar : StateVar/StateVar  TriggerInit=[490 139 605 201]  StateName=PreSlew
      settings: SourceProductName=Bose Talaria
  TSP : TSP/TSP  TriggerInit=[110 134 215 206]  TspName=PreSlew  IfDefMacro=IfdefMacro  Role=Automatic
      settings: SourceProductName=Bose Talaria
  TrivialInterpretation : StateVar/TrivialInterpretation  TriggerInit=[330 148 380 192]
      settings: SourceProductName=Bose Talaria
  wires:
  TSP/1 -> TrivialInterpretation/1
  TrivialInterpretation/1 -> StateVar/1

== system Model_InterpretationEngine64/ModelPreAmp/DecRate/AudioPilot35/Audiopilot_3_5/NoiseEstimationVariant/RegularNoiseEstimation/RatioCalculation/UpdateFlag ==
  StateVar : StateVar/StateVar  TriggerInit=[490 139 605 201]  StateName=UpdateFlag
      settings: SourceProductName=Bose Talaria
  TSP : TSP/TSP  TriggerInit=[110 134 215 206]  TspName=UpdateFlag  IfDefMacro=IfdefMacro  Role=Automatic
      settings: SourceProductName=Bose Talaria
  TrivialInterpretation : StateVar/TrivialInterpretation  TriggerInit=[330 148 380 192]
      settings: SourceProductName=Bose Talaria
  wires:
  TSP/1 -> TrivialInterpretation/1
  TrivialInterpretation/1 -> StateVar/1

== system Model_InterpretationEngine64/ModelPreAmp/DecRate/Medusa5H1/MedusaHoligram/Medusa5H1 Part 1/CAE Treble Boost/Audio Passthrough/Target StateVar ==
  StateVar : StateVar/StateVar  TriggerInit=[490 139 605 201]  StateName=DummyState
      settings: SourceProductName=Bose Talaria
  TSP : TSP/TSP  TriggerInit=[110 134 215 206]  TspName=DummyState  IfDefMacro=IfdefMacro  Role=Automatic
      settings: SourceProductName=Bose Talaria
  TrivialInterpretation : StateVar/TrivialInterpretation  TriggerInit=[330 148 380 192]
      settings: SourceProductName=Bose Talaria
  wires:
  TrivialInterpretation/1 -> StateVar/1
  TSP/1 -> TrivialInterpretation/1

== system Model_InterpretationEngine64/ModelPreAmp/DecRate/Medusa5H1/MedusaHoligram/Medusa5H1 Part 2/Mono Detector/Mono Detector/Target StateVar ==
  StateVar : StateVar/StateVar  TriggerInit=[490 139 605 201]  StateName=LevelCenter
      settings: SourceProductName=Bose Talaria
  TSP : TSP/TSP  TriggerInit=[110 134 215 206]  TspName=LevelCenter  IfDefMacro=IfdefMacro  Role=Automatic
      settings: SourceProductName=Bose Talaria
  TrivialInterpretation : StateVar/TrivialInterpretation  TriggerInit=[330 148 380 192]
      settings: SourceProductName=Bose Talaria
  wires:
  TrivialInterpretation/1 -> StateVar/1
  TSP/1 -> TrivialInterpretation/1

== system Model_InterpretationEngine64/ModelPreAmp/DecRate/AudioPilot35/Audiopilot_3_5/NoiseEstimationVariant/RegularNoiseEstimation/HFNoiseEstimatorCoh/HfNoiseMusicSeparation /MicPsdLevel ==
  TargetStateVar : Subsystem  mask(Talaria Target State Variable){TriggerInit=[-280 -89 -140 -21], TspName=MicPsdLevel, StateName=MicPsdLevel, UseSameName=on, IfdefMacro=[]}
      mask prompts: TriggerInit "Hidden: MoveFcn redraw"; TspName "Name:"; StateName "Name of StateVar:"; UseSameName "Use same name for state variable and TSP"; IfdefMacro "Additional #ifdef macro to enable trigger capture:"
      mask help: The TargetStateVar block encapsultes a Target State Probe (TSP), a State Variable, and a Trivial Interpretation between them.
      mask init:
      | [ok,tspPath,activeStatePath] = TargetStateVarMask.Init(gcbh);
      settings: MoveFcn=TargetStateVarMask.CB_TriggerInit(gcbh);
      mask Help: See help for StateVar and TSP blocks
      mask Callback TriggerInit: TargetStateVarMask.CB_TriggerInit(gcbh);
      mask TypeOptions TspName: TSP/TspName
      mask TypeOptions StateName: StateVar/StateName
      mask Callback UseSameName: TargetStateVarMask.CB_UseSameName(gcbh);
      mask TypeOptions IfdefMacro: TSP/IfdefMacro
      mask DialogControl AdvancedPanel Prompt: Advanced
      mask DialogControl ConvertToFullInterpretation Prompt: Irreversible conversion to full interpretation
      mask DialogControl ConvertToFullInterpretation Callback: TargetStateVarMask.CB_ConvertToFullInterpretation(gcbh);
      mask DialogControl ErrorContainer Prompt: Error Messages
      mask Display:
      | % retrieve icon definition
      | [path,w,h] = TargetStateVarMask.Icon();
      | 
      | % retrieve the block's pixel size
      | pos = get(gcbh,'position');
      | bw = pos(3) - pos(1);
      | bh = pos(4) - pos(2);
      | 
      | % draw centered icon
      | xAdj = bw/2 - w/2 + 5;
      | yAdj = bh/2 - h/2 + 4;
      | for i=1:length(path)
      | 	patch(path(i).x+xAdj, path(i).y+yAdj, path(i).rgb);
      | end
      | 
      | % show the top name or an X
      | if (exist('ok','var') && ok)
      | 	text(bw*0.5, bh*0.2, tspPath, 'horizontalAlignment', 'center');
      | 	patch(0,0,[1 1 1]);
      | 	patch(bw,bh,[1 1 1]);
      | else
      | 	tx=bw*0.03;
      | 	ty=bh*0.03;
      | 	patch([0 tx bw bw-tx], [ty 0 bh-ty bh], [1 0 0]);
      | 	patch([0 bw-tx bw tx], [bh-ty 0 ty bh], [1 0 0]);
      | end

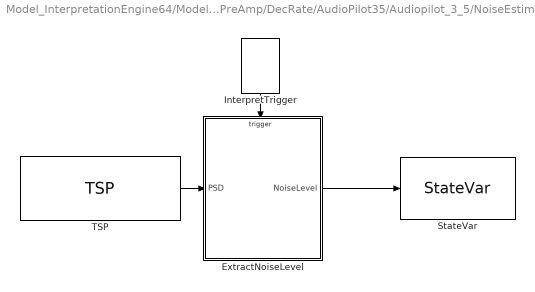
== system Model_InterpretationEngine64/ModelPreAmp/DecRate/AudioPilot35/Audiopilot_3_5/NoiseEstimationVariant/RegularNoiseEstimation/HFNoiseEstimatorCoh/HfNoiseMusicSeparation /NoisePsdLevel ==
  ExtractNoiseLevel : MATLAB Function  TreatAsAtomicUnit=on  mask(Talaria Interpretation){}
      mask help: This MATLAB Function Block can be automatically inserted by several automation routines. Once placed, the block is ready to accept interpretation logic from the model designer.
  InterpretTrigger : StateVar/InterpretTrigger  TriggerInit=[331 20 369 75]
      settings: SourceProductName=Bose Talaria
  StateVar : StateVar/StateVar  TriggerInit=[490 139 605 201]  StateName=NoisePsdLevel
      settings: SourceProductName=Bose Talaria
  TSP : TSP/TSP  TriggerInit=[110 138 270 202]  TspName=PowerSpectralDensity  IfDefMacro=[]  Role=Automatic
      settings: SourceProductName=Bose Talaria
  wires:
  TSP/1 -> ExtractNoiseLevel/1(PSD)
  InterpretTrigger/1 -> ExtractNoiseLevel/Trigger
  ExtractNoiseLevel/1(NoiseLevel) -> StateVar/1

== system Model_InterpretationEngine64/ModelPreAmp/DecRate/AudioPilot35/Audiopilot_3_5/NoiseEstimationVariant/RegularNoiseEstimation/HFNoiseEstimatorCoh/PostProcessing/HfImpulseRejection ==
  note: Impulse and Speech Rejection
  FeaturePath : FeaturePath/FeaturePath  FeatureName=ImpulseRejection  IsGroup=off  GroupNumber=-1  IsModule=off  TriggerInit=[750 304 1100 406]
      settings: SourceProductName=Bose Talaria
  MinSearch : Subsystem
  Pmin : Subsystem  mask(Talaria Target State Variable){TriggerInit=[1015 256 1155 324], TspName=Pmin, StateName=Pmin, UseSameName=on, IfdefMacro=[]}
      mask prompts: TriggerInit "Hidden: MoveFcn redraw"; TspName "Name:"; StateName "Name of StateVar:"; UseSameName "Use same name for state variable and TSP"; IfdefMacro "Additional #ifdef macro to enable trigger capture:"
      mask help: The TargetStateVar block encapsultes a Target State Probe (TSP), a State Variable, and a Trivial Interpretation between them.
      mask init:
      | [ok,tspPath,activeStatePath] = TargetStateVarMask.Init(gcbh);
      settings: MoveFcn=TargetStateVarMask.CB_TriggerInit(gcbh);
      mask Help: See help for StateVar and TSP blocks
      mask Callback TriggerInit: TargetStateVarMask.CB_TriggerInit(gcbh);
      mask TypeOptions TspName: TSP/TspName
      mask TypeOptions StateName: StateVar/StateName
      mask Callback UseSameName: TargetStateVarMask.CB_UseSameName(gcbh);
      mask TypeOptions IfdefMacro: TSP/IfdefMacro
      mask DialogControl AdvancedPanel Prompt: Advanced
      mask DialogControl ConvertToFullInterpretation Prompt: Irreversible conversion to full interpretation
      mask DialogControl ConvertToFullInterpretation Callback: TargetStateVarMask.CB_ConvertToFullInterpretation(gcbh);
      mask DialogControl ErrorContainer Prompt: Error Messages
      mask Display:
      | % retrieve icon definition
      | [path,w,h] = TargetStateVarMask.Icon();
      | 
      | % retrieve the block's pixel size
      | pos = get(gcbh,'position');
      | bw = pos(3) - pos(1);
      | bh = pos(4) - pos(2);
      | 
      | % draw centered icon
      | xAdj = bw/2 - w/2 + 5;
      | yAdj = bh/2 - h/2 + 4;
      | for i=1:length(path)
      | 	patch(path(i).x+xAdj, path(i).y+yAdj, path(i).rgb);
      | end
      | 
      | % show the top name or an X
      | if (exist('ok','var') && ok)
      | 	text(bw*0.5, bh*0.2, tspPath, 'horizontalAlignment', 'center');
      | 	patch(0,0,[1 1 1]);
      | 	patch(bw,bh,[1 1 1]);
      | else
      | 	tx=bw*0.03;
      | 	ty=bh*0.03;
      | 	patch([0 tx bw bw-tx], [ty 0 bh-ty bh], [1 0 0]);
      | 	patch([0 bw-tx bw tx], [bh-ty 0 ty bh], [1 0 0]);
      | end

== system Model_InterpretationEngine64/ModelPreAmp/DecRate/AudioPilot35/Audiopilot_3_5/NoiseEstimationVariant/RegularNoiseEstimation/HFNoiseEstimatorCoh/PostProcessing/PostSlew ==
  StateVar : StateVar/StateVar  TriggerInit=[490 139 605 201]  StateName=PostSlew
      settings: SourceProductName=Bose Talaria
  TSP : TSP/TSP  TriggerInit=[110 134 215 206]  TspName=PostSlew  IfDefMacro=IfdefMacro  Role=Automatic
      settings: SourceProductName=Bose Talaria
  TrivialInterpretation : StateVar/TrivialInterpretation  TriggerInit=[330 148 380 192]
      settings: SourceProductName=Bose Talaria
  wires:
  TSP/1 -> TrivialInterpretation/1
  TrivialInterpretation/1 -> StateVar/1

== system Model_InterpretationEngine64/ModelPreAmp/DecRate/AudioPilot35/Audiopilot_3_5/NoiseEstimationVariant/RegularNoiseEstimation/HFNoiseEstimatorCoh/PostProcessing/PreSlew ==
  StateVar : StateVar/StateVar  TriggerInit=[490 139 605 201]  StateName=PreSlew
      settings: SourceProductName=Bose Talaria
  TSP : TSP/TSP  TriggerInit=[110 134 215 206]  TspName=PreSlew  IfDefMacro=IfdefMacro  Role=Automatic
      settings: SourceProductName=Bose Talaria
  TrivialInterpretation : StateVar/TrivialInterpretation  TriggerInit=[330 148 380 192]
      settings: SourceProductName=Bose Talaria
  wires:
  TSP/1 -> TrivialInterpretation/1
  TrivialInterpretation/1 -> StateVar/1

== system Model_InterpretationEngine64/ModelPreAmp/DecRate/AudioPilot35/Audiopilot_3_5/NoiseEstimationVariant/RegularNoiseEstimation/LFNoiseEstimatorCoh/LfNoiseImpulseRejection/FilterOut ==
  StateVar : StateVar/StateVar  TriggerInit=[490 139 605 201]  StateName=FilterOut
      settings: SourceProductName=Bose Talaria
  TSP : TSP/TSP  TriggerInit=[110 134 215 206]  TspName=FilterOut  IfDefMacro=IfdefMacro  Role=Automatic
      settings: SourceProductName=Bose Talaria
  TrivialInterpretation : StateVar/TrivialInterpretation  TriggerInit=[330 148 380 192]
      settings: SourceProductName=Bose Talaria
  wires:
  TSP/1 -> TrivialInterpretation/1
  TrivialInterpretation/1 -> StateVar/1

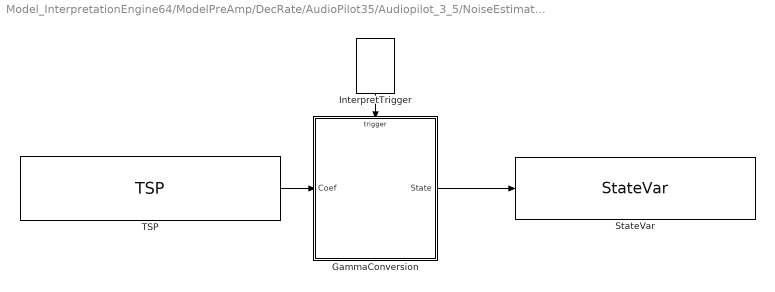
== system Model_InterpretationEngine64/ModelPreAmp/DecRate/AudioPilot35/Audiopilot_3_5/NoiseEstimationVariant/RegularNoiseEstimation/LFNoiseEstimatorCoh/LfNoiseImpulseRejection/GammaTauS ==
  GammaConversion : MATLAB Function  TreatAsAtomicUnit=on
  InterpretTrigger : StateVar/InterpretTrigger  TriggerInit=[336 20 374 75]
      settings: SourceProductName=Bose Talaria
  StateVar : StateVar/StateVar  TriggerInit=[495 139 735 201]  StateName=GammaTauS
      settings: SourceProductName=Bose Talaria
  TSP : TSP/TSP  TriggerInit=[0 138 260 202]  TspName=FiltCoef  IfDefMacro=[]  Role=Automatic
      settings: SourceProductName=Bose Talaria
  wires:
  InterpretTrigger/1 -> GammaConversion/Trigger
  TSP/1 -> GammaConversion/1(Coef)
  GammaConversion/1(State) -> StateVar/1

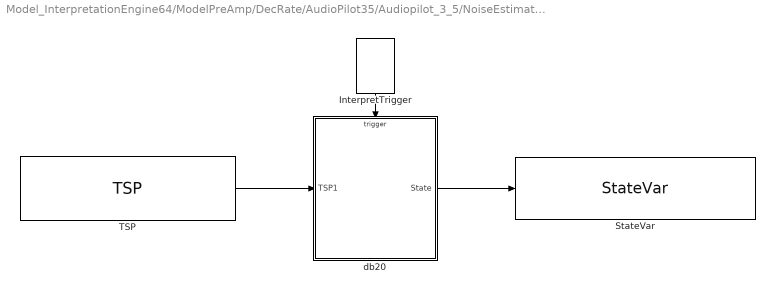
== system Model_InterpretationEngine64/ModelPreAmp/DecRate/AudioPilot35/Audiopilot_3_5/NoiseEstimationVariant/RegularNoiseEstimation/LFNoiseEstimatorCoh/LfNoiseImpulseRejection/ImpulseVariance ==
  InterpretTrigger : StateVar/InterpretTrigger  TriggerInit=[336 20 374 75]
      settings: SourceProductName=Bose Talaria
  StateVar : StateVar/StateVar  TriggerInit=[495 139 735 201]  StateName=ImpulseVarianceDb
      settings: SourceProductName=Bose Talaria
  TSP : TSP/TSP  TriggerInit=[0 138 215 202]  TspName=ImpulseVariance  IfDefMacro=[]  Role=Automatic
      settings: SourceProductName=Bose Talaria
  db20 : MATLAB Function  TreatAsAtomicUnit=on
  wires:
  db20/1(State) -> StateVar/1
  TSP/1 -> db20/1(TSP1)
  InterpretTrigger/1 -> db20/Trigger

== system Model_InterpretationEngine64/ModelPreAmp/DecRate/AudioPilot35/Audiopilot_3_5/NoiseEstimationVariant/RegularNoiseEstimation/LFNoiseEstimatorCoh/LfNoiseImpulseRejection/MusicVariance ==
  InterpretTrigger : StateVar/InterpretTrigger  TriggerInit=[336 20 374 75]
      settings: SourceProductName=Bose Talaria
  StateVar : StateVar/StateVar  TriggerInit=[455 136 685 204]  StateName=MusicVarianceDb
      settings: SourceProductName=Bose Talaria
  TSP : TSP/TSP  TriggerInit=[20 136 260 204]  TspName=MusicVariance  IfDefMacro=[]  Role=Automatic
      settings: SourceProductName=Bose Talaria
  "db20 " : MATLAB Function  TreatAsAtomicUnit=on
  wires:
  "db20 "/1(State) -> StateVar/1
  TSP/1 -> "db20 "/1(TSP1)
  InterpretTrigger/1 -> "db20 "/Trigger

== system Model_InterpretationEngine64/ModelPreAmp/DecRate/AudioPilot35/Audiopilot_3_5/NoiseEstimationVariant/RegularNoiseEstimation/LFNoiseEstimatorCoh/LfNoiseImpulseRejection/NoiseVariance ==
  InterpretTrigger : StateVar/InterpretTrigger  TriggerInit=[336 20 374 75]
      settings: SourceProductName=Bose Talaria
  StateVar : StateVar/StateVar  TriggerInit=[455 136 685 204]  StateName=NoiseVarianceDb
      settings: SourceProductName=Bose Talaria
  TSP : TSP/TSP  TriggerInit=[20 136 260 204]  TspName=NoiseVariance  IfDefMacro=[]  Role=Automatic
      settings: SourceProductName=Bose Talaria
  "db20 " : MATLAB Function  TreatAsAtomicUnit=on
  wires:
  InterpretTrigger/1 -> "db20 "/Trigger
  TSP/1 -> "db20 "/1(TSP1)
  "db20 "/1(State) -> StateVar/1

== system Model_InterpretationEngine64/ModelPreAmp/DecRate/AudioPilot35/Audiopilot_3_5/NoiseEstimationVariant/RegularNoiseEstimation/LFNoiseEstimatorCoh/LfNoiseImpulseRejection/TotalVariance ==
  InterpretTrigger : StateVar/InterpretTrigger  TriggerInit=[336 20 374 75]
      settings: SourceProductName=Bose Talaria
  StateVar : StateVar/StateVar  TriggerInit=[455 136 685 204]  StateName=TotalVarianceDb
      settings: SourceProductName=Bose Talaria
  TSP : TSP/TSP  TriggerInit=[20 136 260 204]  TspName=TotalVariance  IfDefMacro=[]  Role=Automatic
      settings: SourceProductName=Bose Talaria
  "db20 " : MATLAB Function  TreatAsAtomicUnit=on
  wires:
  InterpretTrigger/1 -> "db20 "/Trigger
  TSP/1 -> "db20 "/1(TSP1)
  "db20 "/1(State) -> StateVar/1
